simulink model "sl_synch"  (Simulink 8.3)
settings: Solver=VariableStepDiscrete  StartTime=0.0  StopTime=inf  MaxStep=.01  RelTol=1e-3
PostLoadFcn:
  | % Load the GUI
  | h_synch_gui = sl_synch_gui;
  | 
  | % Adjust its position
  | set(h_synch_gui,'Position',[74.4 28 63 18.08])
StartFcn:
  | % The user may have closed the GUI
  | try
  | 
  | % Get the string of the startstop pushbutton.
  | mystring = get(findobj(h_synch_gui,'Tag','pushbutton_startstop'),'String');
  | 
  | % See if the string is "Start Simulation."
  | % If it is, that implies that the start wasn't driven by the GUI.
  | % Thus we need to update the GUI by making a callback to the startstop function.
  | if strcmp(mystring,'Start Simulation')
  |   sl_synch_gui('pushbutton_startstop_Callback',startstop_hObject,[],sl_synch_handles)
  | end
  | 
  | end
StopFcn:
  | % The user may have closed the GUI
  | try
  | 
  | % Get the string of the startstop pushbutton.
  | mystring = get(findobj(h_synch_gui,'Tag','pushbutton_startstop'),'String');
  | 
  | % See if the string is "Stop Simulation."
  | % If it is, that implies that the stop wasn't driven by the GUI.
  | % Thus we need to update the GUI by making a callback to the startstop function.
  | if strcmp(mystring,'Stop Simulation')
  |   sl_synch_gui('pushbutton_startstop_Callback',startstop_hObject,[],sl_synch_handles)
  | end
  | 
  | end
CloseFcn:
  | % Try to close the GUI
  | % The user might have already closed it.
  | try
  |   close(h_synch_gui)
  | end
settings Model: Creator=wcampbel  LastModifiedBy=Maryam
settings OptimizationCC: ExpressionDepthLimit=2147483647
settings DebuggingCC: FcnCallInpInsideContextMsg=UseLocalSettings

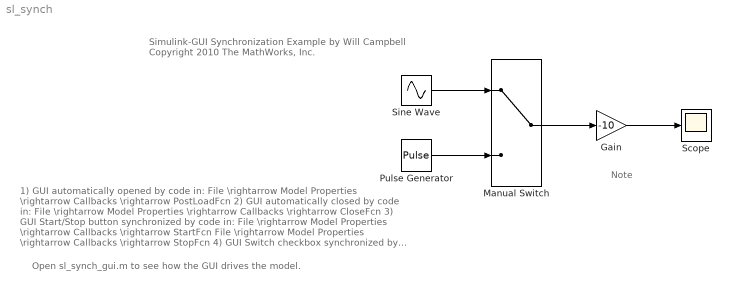
== system sl_synch ==
  note: Simulink-GUI Synchronization Example
      | by Will Campbell
      | Copyright 2010 The MathWorks, Inc.
  note: 1) GUI automatically opened by code in:
      |      File \rightarrow Model Properties \rightarrow Callbacks \rightarrow PostLoadFcn
      | 2) GUI automatically closed by code in:
      |      File \rightarrow Model Properties \rightarrow Callbacks \rightarrow CloseFcn
      | 3) GUI Start/Stop button synchronized by code in:
      |      File \rightarrow Model Properties \rightarrow Callbacks \rightarrow StartFcn
      |      File \rightarrow Model Properties \rightarrow Callbacks \rightarrow StopFcn
      | 4) GUI Switch checkbox synchronized by code in:
      |      Manual Switch \rightarrow Block Properties \rightarrow Callbacks \rightarrow OpenFcn
  note: Open sl_synch_gui.m to see how the GUI drives the model.
  note: Note
  Gain : Gain  Gain=-10
  Manual Switch : ManualSwitch
  Pulse Generator : DiscretePulseGenerator  PulseType=Time based  Period=2.5  PulseWidth=25  PhaseDelay=3
  Scope : Scope
      settings: TimeRange=10  YMin=-10  YMax=10
  Sine Wave : Sin  SampleTime=0
  wires:
  Sine Wave/1 -> Manual Switch/1
  Manual Switch/1 -> Gain/1
  Gain/1 -> Scope/1
  Pulse Generator/1 -> Manual Switch/2
